simulink model "soc_dvbs2_fpga"  (R2025b)
settings: Solver=FixedStepDiscrete  StartTime=0.0  StopTime=0  RelTol=1e-3
InitFcn:
  | soc_dvbs2_init;
values from neighbouring files (symbols this model uses):
  Rsym = 4e6    (= 4000000)    [soc_dvbs2_init.m]
  soc_dvbs2_txPacketBits = [1 1 0 1 0 1 1 1 0 1 1 1 ... (2972 elements, 2972x1)]    [soc_dvbs2_txPacketBits.mat]
  syncWord = (dec2bin(hex2dec('AC')) - '0').'    [soc_dvbs2_init.m]
  txDataOut = txobj(frameBits(:))    [soc_dvbs2_init.m]
  txFiltCoeff = txobj.pTxFilterCoeff    [soc_dvbs2_init.m]
undefined symbols (not defined in the file or in its folder): Add, coefficientsLog, coefficientsSqrt1, coefficientsSqrt2, dataBits, designMultirateFIR, noisePow, NumBits1, NumBits2, seedsURNG1, seedsURNG2, Shift, Slope1, Slope2, soc_dvbs2_designFIRFilter, txDataOutS1, txDataOutS10, txDataOutS12, txDataOutS13, txDataOutS14, txDataOutS15, txDataOutS16, txDataOutS18, txDataOutS19, txDataOutS2, txDataOutS20, txDataOutS21, txDataOutS22, txDataOutS24, txDataOutS25, txDataOutS26, txDataOutS27, txDataOutS3, txDataOutS4, txDataOutS5, txDataOutS6, txDataOutS7, txDataOutS8, txDataOutS9
libraries: simulink x214, hdlsllib x211, dspsigops x22, dsphdlfiltering2 x8, dsphdlsigops2 x5, commseqgen3 x5, dsphdlmathfun2 x3, hwlogicconnlib x2, whdledac x2, commhdlcrc x2, whdlutilities x1, whdlmod x1
(part 6 of 12)

== system soc_dvbs2_fpga/DVBS2/DVBS2 TxRx/DVB-S2 HDL Receiver/Stream Recovery/BB Decoder/Extract BBHeader/Extract MATYPE1 ==
  bitsIn : Inport
  idx : Inport  Port=2
  validIn : Inport  Port=3
  Bit Concat : hdlsllib/Logic and Bit Operations/Bit Concat  numInputs=2
  Bit Concat1 : hdlsllib/Logic and Bit Operations/Bit Concat  numInputs=2
  Compare To Constant : simulink/Logic and Bit Operations/Compare To Constant  relop===  const=0  OutDataTypeStr=boolean
  Compare To Constant1 : simulink/Logic and Bit Operations/Compare To Constant  relop===  const=1  OutDataTypeStr=boolean
  Compare To Constant2 : simulink/Logic and Bit Operations/Compare To Constant  relop===  const=2  OutDataTypeStr=boolean
  Compare To Constant3 : simulink/Logic and Bit Operations/Compare To Constant  relop===  const=3  OutDataTypeStr=boolean
  Compare To Constant4 : simulink/Logic and Bit Operations/Compare To Constant  relop===  const=4  OutDataTypeStr=boolean
  Compare To Constant5 : simulink/Logic and Bit Operations/Compare To Constant  relop===  const=5  OutDataTypeStr=boolean
  Compare To Constant6 : simulink/Logic and Bit Operations/Compare To Constant  relop===  const=6  OutDataTypeStr=boolean
  Compare To Constant7 : simulink/Logic and Bit Operations/Compare To Constant  relop===  const=7  OutDataTypeStr=boolean
  Delay{,1..6} (7 alike) : Delay  DelayLength=1
  Logical Operator{,1..7} (8 alike) : Logic  AllPortsSameDT=off  OutDataTypeStr=boolean
  Unit Delay Enabled Synchronous{,1..7} (8 alike) : hdlsllib/Discrete/Unit Delay Enabled Synchronous  InitialCondition=0.0  SampleTime=-1
  TSorGS : Outport
  SISorMIS : Outport  Port=2
  CCMorACM : Outport  Port=3
  ISSYI : Outport  Port=4
  NPD : Outport  Port=5
  RO : Outport  Port=6
  wires:
  Delay6/1 -> Unit Delay Enabled Synchronous7/2
  Unit Delay Enabled Synchronous7/1 -> RO/1
  Logical Operator7/1 -> Delay6/1
  Bit Concat1/1 -> Unit Delay Enabled Synchronous7/1
  Unit Delay Enabled Synchronous6/1 -> Bit Concat1/1
  validIn/1 -> Logical Operator/2, Logical Operator3/2, Logical Operator4/2, Logical Operator5/2, Logical Operator6/2, Logical Operator7/2, Logical Operator2/2, Logical Operator1/2
  Compare To Constant7/1 -> Logical Operator7/1
  Compare To Constant6/1 -> Logical Operator6/1
  Logical Operator6/1 -> Unit Delay Enabled Synchronous6/2
  Unit Delay Enabled Synchronous5/1 -> NPD/1
  Delay5/1 -> Unit Delay Enabled Synchronous5/2
  Logical Operator5/1 -> Delay5/1
  Compare To Constant5/1 -> Logical Operator5/1
  Unit Delay Enabled Synchronous1/1 -> TSorGS/1
  Unit Delay Enabled Synchronous4/1 -> ISSYI/1
  Logical Operator/1 -> Unit Delay Enabled Synchronous/2
  Compare To Constant3/1 -> Logical Operator3/1
  Delay/1 -> Unit Delay Enabled Synchronous1/2
  Logical Operator2/1 -> Delay2/1
  Logical Operator3/1 -> Delay3/1
  Compare To Constant/1 -> Logical Operator/1
  Compare To Constant4/1 -> Logical Operator4/1
  Delay2/1 -> Unit Delay Enabled Synchronous2/2
  bitsIn/1 -> Unit Delay Enabled Synchronous/1, Delay1/1, Unit Delay Enabled Synchronous6/1
  Delay4/1 -> Unit Delay Enabled Synchronous4/2
  Delay1/1 -> Bit Concat/2, Unit Delay Enabled Synchronous2/1, Unit Delay Enabled Synchronous3/1, Unit Delay Enabled Synchronous4/1, Unit Delay Enabled Synchronous5/1, Bit Concat1/2
  Bit Concat/1 -> Unit Delay Enabled Synchronous1/1
  Logical Operator4/1 -> Delay4/1
  idx/1 -> Compare To Constant/1, Compare To Constant1/1, Compare To Constant2/1, Compare To Constant3/1, Compare To Constant5/1, Compare To Constant6/1, Compare To Constant7/1, Compare To Constant4/1
  Compare To Constant1/1 -> Logical Operator1/1
  Unit Delay Enabled Synchronous3/1 -> CCMorACM/1
  Logical Operator1/1 -> Delay/1
  Delay3/1 -> Unit Delay Enabled Synchronous3/2
  Unit Delay Enabled Synchronous/1 -> Bit Concat/1
  Unit Delay Enabled Synchronous2/1 -> SISorMIS/1
  Compare To Constant2/1 -> Logical Operator2/1

== system soc_dvbs2_fpga/DVBS2/DVBS2 TxRx/DVB-S2 HDL Receiver/Stream Recovery/BB Decoder/Extract BBHeader/Extract MATYPE2 ==
  bitsIn : Inport
  idx : Inport  Port=2
  validIn : Inport  Port=3
  Add : Sum  Inputs=|++  OutDataTypeStr=Inherit: Same as first input
  Compare To Constant : simulink/Logic and Bit Operations/Compare To Constant  relop=>=  const=8  OutDataTypeStr=boolean
  Compare To Constant1 : simulink/Logic and Bit Operations/Compare To Constant  relop=<=  const=8+7  OutDataTypeStr=boolean
  Compare To Constant2 : simulink/Logic and Bit Operations/Compare To Constant  relop===  const=16  OutDataTypeStr=boolean
  Data Type Conversion : DataTypeConversion  OutDataTypeStr=uint8  SaturateOnIntegerOverflow=off  RndMeth=Floor
  Gain : Gain  Gain=2  ParamDataTypeStr=fixdt(0,2,0)  OutDataTypeStr=Inherit: Same as input
  Logical Operator : Logic  Inputs=3  AllPortsSameDT=off  OutDataTypeStr=boolean
  Logical Operator1 : Logic  AllPortsSameDT=off  OutDataTypeStr=boolean
  Unit Delay Enabled Synchronous : hdlsllib/Discrete/Unit Delay Enabled Synchronous  InitialCondition=0.0  SampleTime=-1
  Unit Delay Enabled Resettable Synchronous : hdlsllib/Discrete/Unit Delay Enabled Resettable Synchronous  InitialCondition=0.0  SampleTime=-1
  MIS_ISI : Outport
  wires:
  bitsIn/1 -> Data Type Conversion/1
  Compare To Constant1/1 -> Logical Operator/2
  Gain/1 -> Add/2
  Unit Delay Enabled Synchronous/1 -> MIS_ISI/1
  Data Type Conversion/1 -> Add/1
  Compare To Constant2/1 -> Logical Operator1/1
  Unit Delay Enabled Resettable Synchronous/1 -> Unit Delay Enabled Synchronous/1, Gain/1
  idx/1 -> Compare To Constant1/1, Compare To Constant2/1, Compare To Constant/1
  Add/1 -> Unit Delay Enabled Resettable Synchronous/1
  Logical Operator/1 -> Unit Delay Enabled Resettable Synchronous/2
  validIn/1 -> Logical Operator1/2, Logical Operator/3
  Logical Operator1/1 -> Unit Delay Enabled Resettable Synchronous/3, Unit Delay Enabled Synchronous/2
  Compare To Constant/1 -> Logical Operator/1

== system soc_dvbs2_fpga/DVBS2/DVBS2 TxRx/DVB-S2 HDL Receiver/Stream Recovery/BB Decoder/Extract BBHeader/Extract SYNC ==
  bitsIn : Inport
  idx : Inport  Port=2
  validIn : Inport  Port=3
  Add : Sum  Inputs=|++  OutDataTypeStr=Inherit: Same as first input
  Compare To Constant : simulink/Logic and Bit Operations/Compare To Constant  relop=>=  const=48  OutDataTypeStr=boolean
  Compare To Constant1 : simulink/Logic and Bit Operations/Compare To Constant  relop=<=  const=48+7  OutDataTypeStr=boolean
  Compare To Constant2 : simulink/Logic and Bit Operations/Compare To Constant  relop===  const=56  OutDataTypeStr=boolean
  Data Type Conversion : DataTypeConversion  OutDataTypeStr=uint8  SaturateOnIntegerOverflow=off  RndMeth=Floor
  Gain : Gain  Gain=2  ParamDataTypeStr=fixdt(0,2,0)  OutDataTypeStr=Inherit: Same as input
  Logical Operator : Logic  Inputs=3  AllPortsSameDT=off  OutDataTypeStr=boolean
  Logical Operator1 : Logic  AllPortsSameDT=off  OutDataTypeStr=boolean
  Unit Delay Enabled Synchronous : hdlsllib/Discrete/Unit Delay Enabled Synchronous  InitialCondition=0.0  SampleTime=-1
  Unit Delay Enabled Resettable Synchronous : hdlsllib/Discrete/Unit Delay Enabled Resettable Synchronous  InitialCondition=0.0  SampleTime=-1
  SYNC : Outport
  wires:
  Compare To Constant/1 -> Logical Operator/1
  Logical Operator1/1 -> Unit Delay Enabled Synchronous/2, Unit Delay Enabled Resettable Synchronous/3
  validIn/1 -> Logical Operator1/2, Logical Operator/3
  Logical Operator/1 -> Unit Delay Enabled Resettable Synchronous/2
  Add/1 -> Unit Delay Enabled Resettable Synchronous/1
  idx/1 -> Compare To Constant2/1, Compare To Constant1/1, Compare To Constant/1
  Unit Delay Enabled Resettable Synchronous/1 -> Gain/1, Unit Delay Enabled Synchronous/1
  Compare To Constant2/1 -> Logical Operator1/1
  Data Type Conversion/1 -> Add/1
  Unit Delay Enabled Synchronous/1 -> SYNC/1
  Gain/1 -> Add/2
  Compare To Constant1/1 -> Logical Operator/2
  bitsIn/1 -> Data Type Conversion/1

== system soc_dvbs2_fpga/DVBS2/DVBS2 TxRx/DVB-S2 HDL Receiver/Stream Recovery/BB Decoder/Extract BBHeader/Extract SYNCD ==
  bitsIn : Inport
  idx : Inport  Port=2
  validIn : Inport  Port=3
  Add : Sum  Inputs=|++  OutDataTypeStr=Inherit: Same as first input
  Compare To Constant : simulink/Logic and Bit Operations/Compare To Constant  relop=>=  const=56  OutDataTypeStr=boolean
  Compare To Constant1 : simulink/Logic and Bit Operations/Compare To Constant  relop=<=  const=56+15  OutDataTypeStr=boolean
  Data Type Conversion : DataTypeConversion  OutDataTypeStr=uint16  SaturateOnIntegerOverflow=off  RndMeth=Floor
  Delay : Delay  DelayLength=1
  Gain : Gain  Gain=2  ParamDataTypeStr=fixdt(0,2,0)  OutDataTypeStr=Inherit: Same as input
  Logical Operator : Logic  Inputs=3  AllPortsSameDT=off  OutDataTypeStr=boolean
  Logical Operator1 : Logic  AllPortsSameDT=off  OutDataTypeStr=boolean
  Unit Delay Enabled Synchronous : hdlsllib/Discrete/Unit Delay Enabled Synchronous  InitialCondition=0.0  SampleTime=-1
  Unit Delay Enabled Resettable Synchronous : hdlsllib/Discrete/Unit Delay Enabled Resettable Synchronous  InitialCondition=0.0  SampleTime=-1
  DFL : Outport
  wires:
  Delay/1 -> Unit Delay Enabled Synchronous/2, Unit Delay Enabled Resettable Synchronous/3
  Compare To Constant/1 -> Logical Operator/1
  Logical Operator1/1 -> Delay/1
  validIn/1 -> Logical Operator1/2, Logical Operator/3
  Logical Operator/1 -> Unit Delay Enabled Resettable Synchronous/2
  Add/1 -> Unit Delay Enabled Resettable Synchronous/1
  idx/1 -> Compare To Constant1/1, Compare To Constant/1
  Unit Delay Enabled Resettable Synchronous/1 -> Gain/1, Unit Delay Enabled Synchronous/1
  Data Type Conversion/1 -> Add/1
  Unit Delay Enabled Synchronous/1 -> DFL/1
  Gain/1 -> Add/2
  Compare To Constant1/1 -> Logical Operator/2, Logical Operator1/1
  bitsIn/1 -> Data Type Conversion/1

== system soc_dvbs2_fpga/DVBS2/DVBS2 TxRx/DVB-S2 HDL Receiver/Stream Recovery/BB Decoder/Extract BBHeader/Extract UPL ==
  bitsIn : Inport
  idx : Inport  Port=2
  validIn : Inport  Port=3
  Add : Sum  Inputs=|++  OutDataTypeStr=Inherit: Same as first input
  Compare To Constant : simulink/Logic and Bit Operations/Compare To Constant  relop=>=  const=16  OutDataTypeStr=boolean
  Compare To Constant1 : simulink/Logic and Bit Operations/Compare To Constant  relop=<=  const=16+15  OutDataTypeStr=boolean
  Compare To Constant2 : simulink/Logic and Bit Operations/Compare To Constant  relop===  const=32  OutDataTypeStr=boolean
  Data Type Conversion : DataTypeConversion  OutDataTypeStr=uint16  SaturateOnIntegerOverflow=off  RndMeth=Floor
  Gain : Gain  Gain=2  ParamDataTypeStr=fixdt(0,2,0)  OutDataTypeStr=Inherit: Same as input
  Logical Operator : Logic  Inputs=3  AllPortsSameDT=off  OutDataTypeStr=boolean
  Logical Operator1 : Logic  AllPortsSameDT=off  OutDataTypeStr=boolean
  Unit Delay Enabled Synchronous : hdlsllib/Discrete/Unit Delay Enabled Synchronous  InitialCondition=0.0  SampleTime=-1
  Unit Delay Enabled Resettable Synchronous : hdlsllib/Discrete/Unit Delay Enabled Resettable Synchronous  InitialCondition=0.0  SampleTime=-1
  UPL : Outport
  wires:
  Compare To Constant/1 -> Logical Operator/1
  Logical Operator1/1 -> Unit Delay Enabled Synchronous/2, Unit Delay Enabled Resettable Synchronous/3
  validIn/1 -> Logical Operator1/2, Logical Operator/3
  Logical Operator/1 -> Unit Delay Enabled Resettable Synchronous/2
  Add/1 -> Unit Delay Enabled Resettable Synchronous/1
  idx/1 -> Compare To Constant2/1, Compare To Constant1/1, Compare To Constant/1
  Unit Delay Enabled Resettable Synchronous/1 -> Gain/1, Unit Delay Enabled Synchronous/1
  Compare To Constant2/1 -> Logical Operator1/1
  Data Type Conversion/1 -> Add/1
  Unit Delay Enabled Synchronous/1 -> UPL/1
  Gain/1 -> Add/2
  Compare To Constant1/1 -> Logical Operator/2
  bitsIn/1 -> Data Type Conversion/1

== system soc_dvbs2_fpga/DVBS2/DVBS2 TxRx/DVB-S2 HDL Receiver/Stream Recovery/BB Decoder/Extract BBHeader/Saturate UPL value ==
  note: if UPL > DFL - 10
      | saturatedUPL = DFL - 10;
      | else
      | saturatedUPL = UPL
      | end
  UPL : Inport
  DFL : Inport  Port=2
  Add : Sum  Inputs=+-  OutDataTypeStr=Inherit: Same as first input
  Constant : Constant  Value=10  OutDataTypeStr=fixdt(0,4,0)  SampleTime=-1
  Relational Operator : RelationalOperator  Operator=>  OutDataTypeStr=boolean  RndMeth=Simplest  InputSameDT=off
  Switch : Switch  Criteria=u2 ~= 0  SaturateOnIntegerOverflow=off  InputSameDT=off
  saturatedUPL : Outport
  wires:
  Constant/1 -> Add/2
  Relational Operator/1 -> Switch/2
  UPL/1 -> Switch/3, Relational Operator/1
  Add/1 -> Relational Operator/2, Switch/1
  DFL/1 -> Add/1
  Switch/1 -> saturatedUPL/1

== system soc_dvbs2_fpga/DVBS2/DVBS2 TxRx/DVB-S2 HDL Receiver/Stream Recovery/BB Decoder/Extract Data Field/Indicate SYNCD bit ==
  rst : Inport
  Distance : Inport  Port=2
  validIn : Inport  Port=3
  Constant1 : Constant  OutDataTypeStr=fixdt(0,1,0)  SampleTime=-1
  Constant2 : Constant  Value=0  OutDataTypeStr=fixdt(0,1,0)  SampleTime=-1
  HDL Counter1 : hdlsllib/Sources/HDL Counter  CountType=Free running  CountInit=0  CountStep=1  CountMax=25  CountFromType=Initial value  CountFrom=0  CountResetPort=on  CountLoadPort=off  CountEnbPort=on  CountDirPort=off  CountHitOutputPort=off  CountDataType=Unsigned  CountWordLen=16  CountFracLen=0  CountSampTime=1
  Logical Operator3 : Logic  AllPortsSameDT=off  OutDataTypeStr=boolean
  Relational Operator1 : RelationalOperator  Operator===  OutDataTypeStr=boolean  RndMeth=Simplest  InputSameDT=off
  Subtract1 : Sum  Inputs=+-  OutDataTypeStr=Inherit: Same as first input
  Switch : Switch  Criteria=u2 ~= 0  SaturateOnIntegerOverflow=off  InputSameDT=off
  trigger : Outport
  wires:
  rst/1 -> HDL Counter1/1
  Logical Operator3/1 -> trigger/1
  Switch/1 -> Subtract1/2
  validIn/1 -> HDL Counter1/2, Logical Operator3/2
  Distance/1 -> Subtract1/1, Switch/2
  Subtract1/1 -> Relational Operator1/1
  Relational Operator1/1 -> Logical Operator3/1
  Constant2/1 -> Switch/3
  Constant1/1 -> Switch/1
  HDL Counter1/1 -> Relational Operator1/2

== system soc_dvbs2_fpga/DVBS2/DVBS2 TxRx/DVB-S2 HDL Receiver/Stream Recovery/BB Decoder/Extract Stream/Extract User Packet  ==
  SYNCD : Inport
  bitsIn : Inport  Port=2
  startIn : Inport  Port=3
  endIn : Inport  Port=4
  validIn : Inport  Port=5
  UPL : Inport  Port=6
  Compare To Constant : simulink/Logic and Bit Operations/Compare To Constant  relop=~=  const=0  OutDataTypeStr=boolean
  Delay{1..2,4..7,9..10,12,19,21} (11 alike) : Delay  DelayLength=1
  Demux : Demux  Outputs=2
  Indicate SYNCD bit : Subsystem
  Logical Operator : Logic  AllPortsSameDT=off  OutDataTypeStr=boolean
  Logical Operator1 : Logic  AllPortsSameDT=off  OutDataTypeStr=boolean
  Logical Operator2 : Logic  Operator=NOT  AllPortsSameDT=off  OutDataTypeStr=boolean
  Logical Operator3 : Logic  Operator=OR  AllPortsSameDT=off  OutDataTypeStr=boolean
  Sample Discard Control : MATLAB Function  TreatAsAtomicUnit=on
  Terminator1 : Terminator
  Variable Count Limited HDL Counter : MATLAB Function  TreatAsAtomicUnit=on
  dataOut : Outport
  startOut : Outport  Port=2
  endOut : Outport  Port=3
  validOut : Outport  Port=4
  invalidPkt : Outport  Port=5
  wires:
  validIn/1 -> Logical Operator/2
  Compare To Constant/1 -> Logical Operator/1
  Demux/2 -> Logical Operator2/1, Logical Operator3/1
  Demux/1 -> startOut/1
  Delay12/1 -> Sample Discard Control/2(startIn)
  Delay10/1 -> dataOut/1
  Delay9/1 -> Sample Discard Control/3(endIn)
  Variable Count Limited HDL Counter/1(Hit) -> Sample Discard Control/1(dataIn)
  Delay21/1 -> Delay6/1
  Logical Operator/1 -> Delay2/1
  UPL/1 -> Delay21/1, Compare To Constant/1
  Delay5/1 -> Sample Discard Control/4(validIn), Variable Count Limited HDL Counter/3(enb)
  Delay6/1 -> Variable Count Limited HDL Counter/2(countToValue)
  Delay7/1 -> Delay9/1
  endIn/1 -> Delay7/1
  Indicate SYNCD bit/1(trigger) -> Delay12/1, Variable Count Limited HDL Counter/1(rst)
  startIn/1 -> Indicate SYNCD bit/1(rst)
  Delay1/1 -> Indicate SYNCD bit/2(Distance)
  Delay4/1 -> Delay10/1
  SYNCD/1 -> Delay1/1
  Delay2/1 -> Delay5/1, Indicate SYNCD bit/3(validIn)
  bitsIn/1 -> Delay19/1
  Delay19/1 -> Delay4/1
  Sample Discard Control/1(dataOut) -> Demux/1
  Sample Discard Control/2(startOut) -> Terminator1/1
  Sample Discard Control/3(endOut) -> Logical Operator3/2, Logical Operator1/2
  Sample Discard Control/4(validOut) -> validOut/1
  Logical Operator1/1 -> invalidPkt/1
  Logical Operator2/1 -> Logical Operator1/1
  Logical Operator3/1 -> endOut/1

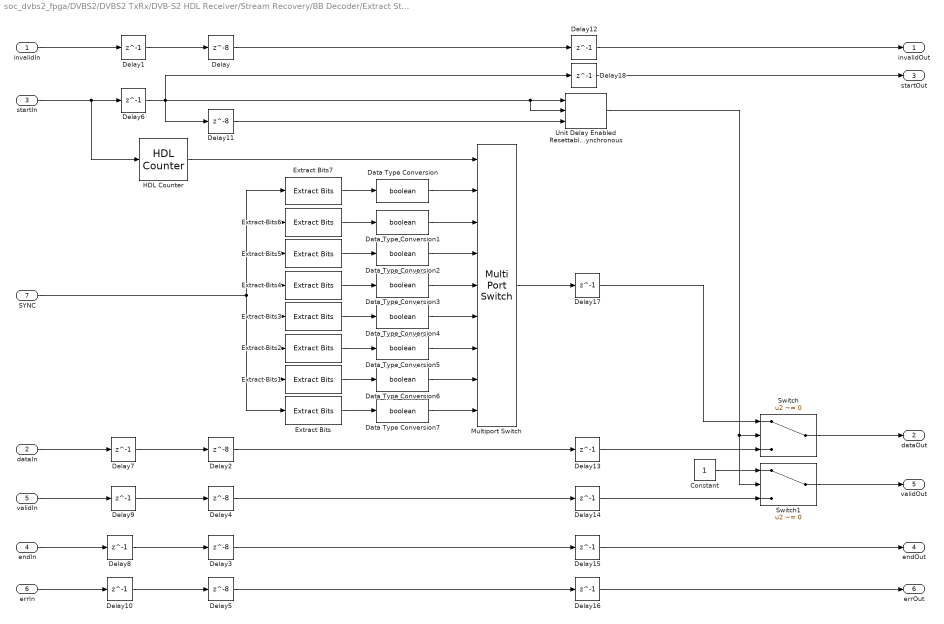
== system soc_dvbs2_fpga/DVBS2/DVBS2 TxRx/DVB-S2 HDL Receiver/Stream Recovery/BB Decoder/Extract Stream/Insert SYNC ==
  invalidIn : Inport
  dataIn : Inport  Port=2
  startIn : Inport  Port=3
  endIn : Inport  Port=4
  validIn : Inport  Port=5
  errIn : Inport  Port=6
  SYNC : Inport  Port=7
  Constant : Constant  OutDataTypeStr=boolean  SampleTime=-1
  Data Type Conversion{,1..7} (8 alike) : DataTypeConversion  OutDataTypeStr=boolean  SaturateOnIntegerOverflow=off  RndMeth=Floor
  Delay{,2..5,11} (6 alike) : Delay  DelayLength=8
  Delay{1,6..10,12..18} (13 alike) : Delay  DelayLength=1
  Extract Bits : simulink/Logic and Bit Operations/Extract Bits  bitsToExtract=Range of bits  numBits=8  bitIdxRange=0  outScalingMode=Treat bit field as an integer
  Extract Bits1 : simulink/Logic and Bit Operations/Extract Bits  bitsToExtract=Range of bits  numBits=8  bitIdxRange=1  outScalingMode=Treat bit field as an integer
  Extract Bits2 : simulink/Logic and Bit Operations/Extract Bits  bitsToExtract=Range of bits  numBits=8  bitIdxRange=2  outScalingMode=Treat bit field as an integer
  Extract Bits3 : simulink/Logic and Bit Operations/Extract Bits  bitsToExtract=Range of bits  numBits=8  bitIdxRange=3  outScalingMode=Treat bit field as an integer
  Extract Bits4 : simulink/Logic and Bit Operations/Extract Bits  bitsToExtract=Range of bits  numBits=8  bitIdxRange=4  outScalingMode=Treat bit field as an integer
  Extract Bits5 : simulink/Logic and Bit Operations/Extract Bits  bitsToExtract=Range of bits  numBits=8  bitIdxRange=5  outScalingMode=Treat bit field as an integer
  Extract Bits6 : simulink/Logic and Bit Operations/Extract Bits  bitsToExtract=Range of bits  numBits=8  bitIdxRange=6  outScalingMode=Treat bit field as an integer
  Extract Bits7 : simulink/Logic and Bit Operations/Extract Bits  bitsToExtract=Range of bits  numBits=8  bitIdxRange=7  outScalingMode=Treat bit field as an integer
  HDL Counter : hdlsllib/Sources/HDL Counter  CountType=Count limited  CountInit=0  CountStep=1  CountMax=7  CountFromType=Initial value  CountFrom=0  CountResetPort=on  CountLoadPort=off  CountEnbPort=off  CountDirPort=off  CountHitOutputPort=off  CountDataType=Unsigned  CountWordLen=3  CountFracLen=0  CountSampTime=1
  Multiport Switch : MultiPortSwitch  DataPortOrder=Zero-based contiguous  Inputs=8  zeroidx=on  SaturateOnIntegerOverflow=off  InputSameDT=off
  Switch : Switch  Criteria=u2 ~= 0  SaturateOnIntegerOverflow=off  InputSameDT=off
  Switch1 : Switch  Criteria=u2 ~= 0  SaturateOnIntegerOverflow=off  InputSameDT=off
  Unit Delay Enabled Resettable Synchronous : hdlsllib/Discrete/Unit Delay Enabled Resettable Synchronous  InitialCondition=0.0  SampleTime=-1
  invalidOut : Outport
  dataOut : Outport  Port=2
  startOut : Outport  Port=3
  endOut : Outport  Port=4
  validOut : Outport  Port=5
  errOut : Outport  Port=6
  wires:
  Switch/1 -> dataOut/1
  Switch1/1 -> validOut/1
  Delay18/1 -> startOut/1
  Delay10/1 -> Delay5/1
  errIn/1 -> Delay10/1
  endIn/1 -> Delay8/1
  Delay14/1 -> Switch1/3
  Data Type Conversion7/1 -> Multiport Switch/9
  Multiport Switch/1 -> Delay17/1
  startIn/1 -> HDL Counter/1, Delay6/1
  Delay2/1 -> Delay13/1
  Delay12/1 -> invalidOut/1
  Data Type Conversion1/1 -> Multiport Switch/3
  Extract Bits4/1 -> Data Type Conversion3/1
  Unit Delay Enabled Resettable Synchronous/1 -> Switch1/2, Switch/2
  Delay6/1 -> Delay18/1, Delay11/1, Unit Delay Enabled Resettable Synchronous/2, Unit Delay Enabled Resettable Synchronous/1
  Data Type Conversion5/1 -> Multiport Switch/7
  Delay1/1 -> Delay/1
  Extract Bits/1 -> Data Type Conversion7/1
  dataIn/1 -> Delay7/1
  Delay7/1 -> Delay2/1
  Delay11/1 -> Unit Delay Enabled Resettable Synchronous/3
  Extract Bits1/1 -> Data Type Conversion6/1
  invalidIn/1 -> Delay1/1
  Delay9/1 -> Delay4/1
  Extract Bits6/1 -> Data Type Conversion1/1
  Data Type Conversion4/1 -> Multiport Switch/6
  Data Type Conversion2/1 -> Multiport Switch/4
  Data Type Conversion3/1 -> Multiport Switch/5
  Extract Bits5/1 -> Data Type Conversion2/1
  Extract Bits7/1 -> Data Type Conversion/1
  Delay5/1 -> Delay16/1
  Data Type Conversion6/1 -> Multiport Switch/8
  Delay16/1 -> errOut/1
  Delay17/1 -> Switch/1
  validIn/1 -> Delay9/1
  HDL Counter/1 -> Multiport Switch/1
  Constant/1 -> Switch1/1
  Delay3/1 -> Delay15/1
  Delay8/1 -> Delay3/1
  Delay/1 -> Delay12/1
  Extract Bits2/1 -> Data Type Conversion5/1
  Delay13/1 -> Switch/3
  Delay15/1 -> endOut/1
  Data Type Conversion/1 -> Multiport Switch/2
  Extract Bits3/1 -> Data Type Conversion4/1
  SYNC/1 -> Extract Bits7/1, Extract Bits6/1, Extract Bits5/1, Extract Bits4/1, Extract Bits/1, Extract Bits1/1, Extract Bits2/1, Extract Bits3/1
  Delay4/1 -> Delay14/1

== system soc_dvbs2_fpga/DVBS2/DVBS2 TxRx/DVB-S2 HDL Receiver/Synchronizer and PL Header Decoder/Fine Phase Synchronizer/Power Q and Beta Offset Rotation/Complex Multiplier ==
  In1 : Inport
  In2 : Inport  Port=2
  AddADn : Sum  Inputs=++|  OutDataTypeStr=Inherit: Inherit via back propagation
  AddAUp : Sum  Inputs=|+-  OutDataTypeStr=Inherit: Inherit via back propagation
  AddBCtr : Sum  Inputs=+|+
  AddBDn : Sum  Inputs=|+-
  AddBUp : Sum  Inputs=++|
  Complex to Real-Imag : ComplexToRealImag
  Complex to Real-Imag1 : ComplexToRealImag
  Data Type Duplicate : DataTypeDuplicate
  Delay{1..8,21} (9 alike) : Delay
  Delay{9..20} (12 alike) : Delay  DelayLength=1
  ProductCtr : Product
  ProductDn : Product
  ProductUp : Product
  Real-Imag to Complex : RealImagToComplex
  Out1 : Outport  VectorParamsAs1DForOutWhenUnconnected=off
  wires:
  In1/1 -> Complex to Real-Imag/1, Data Type Duplicate/1
  In2/1 -> Complex to Real-Imag1/1
  Complex to Real-Imag1/1 -> [RE2]
  Complex to Real-Imag1/2 -> [IM2]
  [IM2] -> Delay10/1
  [RE2] -> Delay9/1
  Complex to Real-Imag/1 -> Delay11/1
  AddBUp/1 -> Delay8/1
  [RE2] -> Delay14/1
  [IM2] -> Delay15/1
  AddBDn/1 -> Delay5/1
  Complex to Real-Imag/2 -> Delay13/1
  AddBCtr/1 -> Delay2/1
  [IM2] -> Delay12/1
  ProductUp/1 -> Delay21/1
  ProductCtr/1 -> Delay7/1
  ProductDn/1 -> Delay6/1
  AddADn/1 -> Delay20/1
  AddAUp/1 -> Delay19/1
  Real-Imag to Complex/1 -> Out1/1, Data Type Duplicate/2
  Delay21/1 -> Delay16/1
  Delay7/1 -> Delay17/1
  Delay6/1 -> Delay18/1
  Delay5/1 -> ProductDn/2
  Delay4/1 -> ProductDn/1
  Delay3/1 -> ProductCtr/2
  Delay2/1 -> ProductCtr/1
  Delay1/1 -> ProductUp/2
  Delay8/1 -> ProductUp/1
  Delay9/1 -> AddBUp/1
  Delay10/1 -> AddBUp/2
  Delay11/1 -> Delay1/1, AddBCtr/1
  Delay12/1 -> Delay3/1
  Delay13/1 -> Delay4/1, AddBCtr/2
  Delay14/1 -> AddBDn/1
  Delay15/1 -> AddBDn/2
  Delay16/1 -> AddAUp/1
  Delay17/1 -> AddADn/1, AddAUp/2
  Delay18/1 -> AddADn/2
  Delay19/1 -> Real-Imag to Complex/1
  Delay20/1 -> Real-Imag to Complex/2

== system soc_dvbs2_fpga/DVBS2/DVBS2 TxRx/DVB-S2 HDL Receiver/Synchronizer and PL Header Decoder/Fine Phase Synchronizer/Power Q and Beta Offset Rotation/Complex Multiplier1 ==
  In1 : Inport
  In2 : Inport  Port=2
  AddADn : Sum  Inputs=++|  OutDataTypeStr=Inherit: Inherit via back propagation
  AddAUp : Sum  Inputs=|+-  OutDataTypeStr=Inherit: Inherit via back propagation
  AddBCtr : Sum  Inputs=+|+
  AddBDn : Sum  Inputs=|+-
  AddBUp : Sum  Inputs=++|
  Complex to Real-Imag : ComplexToRealImag
  Complex to Real-Imag1 : ComplexToRealImag
  Data Type Duplicate : DataTypeDuplicate
  Delay{1..8,21} (9 alike) : Delay
  Delay{9..20} (12 alike) : Delay  DelayLength=1
  ProductCtr : Product
  ProductDn : Product
  ProductUp : Product
  Real-Imag to Complex : RealImagToComplex
  Out1 : Outport  VectorParamsAs1DForOutWhenUnconnected=off
  wires:
  Delay20/1 -> Real-Imag to Complex/2
  Delay19/1 -> Real-Imag to Complex/1
  Delay18/1 -> AddADn/2
  Delay17/1 -> AddAUp/2, AddADn/1
  Delay16/1 -> AddAUp/1
  Delay15/1 -> AddBDn/2
  Delay14/1 -> AddBDn/1
  Delay13/1 -> AddBCtr/2, Delay4/1
  Delay12/1 -> Delay3/1
  Delay11/1 -> AddBCtr/1, Delay1/1
  Delay10/1 -> AddBUp/2
  Delay9/1 -> AddBUp/1
  Delay8/1 -> ProductUp/1
  Delay1/1 -> ProductUp/2
  Delay2/1 -> ProductCtr/1
  Delay3/1 -> ProductCtr/2
  Delay4/1 -> ProductDn/1
  Delay5/1 -> ProductDn/2
  Delay6/1 -> Delay18/1
  Delay7/1 -> Delay17/1
  Delay21/1 -> Delay16/1
  Real-Imag to Complex/1 -> Data Type Duplicate/2, Out1/1
  AddAUp/1 -> Delay19/1
  AddADn/1 -> Delay20/1
  ProductDn/1 -> Delay6/1
  ProductCtr/1 -> Delay7/1
  ProductUp/1 -> Delay21/1
  [IM2] -> Delay12/1
  AddBCtr/1 -> Delay2/1
  Complex to Real-Imag/2 -> Delay13/1
  AddBDn/1 -> Delay5/1
  [IM2] -> Delay15/1
  [RE2] -> Delay14/1
  AddBUp/1 -> Delay8/1
  Complex to Real-Imag/1 -> Delay11/1
  [RE2] -> Delay9/1
  [IM2] -> Delay10/1
  Complex to Real-Imag1/2 -> [IM2]
  Complex to Real-Imag1/1 -> [RE2]
  In2/1 -> Complex to Real-Imag1/1
  In1/1 -> Data Type Duplicate/1, Complex to Real-Imag/1

== system soc_dvbs2_fpga/DVBS2/DVBS2 TxRx/DVB-S2 HDL Receiver/Synchronizer and PL Header Decoder/Fine Phase Synchronizer/Power Q and Beta Offset Rotation/Complex Multiplier2 ==
  In1 : Inport
  In2 : Inport  Port=2
  AddADn : Sum  Inputs=++|  OutDataTypeStr=Inherit: Inherit via back propagation
  AddAUp : Sum  Inputs=|+-  OutDataTypeStr=Inherit: Inherit via back propagation
  AddBCtr : Sum  Inputs=+|+
  AddBDn : Sum  Inputs=|+-
  AddBUp : Sum  Inputs=++|
  Complex to Real-Imag : ComplexToRealImag
  Complex to Real-Imag1 : ComplexToRealImag
  Data Type Duplicate : DataTypeDuplicate
  Delay{1..8,21} (9 alike) : Delay
  Delay{9..20} (12 alike) : Delay  DelayLength=1
  ProductCtr : Product
  ProductDn : Product
  ProductUp : Product
  Real-Imag to Complex : RealImagToComplex
  Out1 : Outport  VectorParamsAs1DForOutWhenUnconnected=off
  wires:
  In1/1 -> Complex to Real-Imag/1, Data Type Duplicate/1
  In2/1 -> Complex to Real-Imag1/1
  Complex to Real-Imag1/1 -> [RE2]
  Complex to Real-Imag1/2 -> [IM2]
  [IM2] -> Delay10/1
  [RE2] -> Delay9/1
  Complex to Real-Imag/1 -> Delay11/1
  AddBUp/1 -> Delay8/1
  [RE2] -> Delay14/1
  [IM2] -> Delay15/1
  AddBDn/1 -> Delay5/1
  Complex to Real-Imag/2 -> Delay13/1
  AddBCtr/1 -> Delay2/1
  [IM2] -> Delay12/1
  ProductUp/1 -> Delay21/1
  ProductCtr/1 -> Delay7/1
  ProductDn/1 -> Delay6/1
  AddADn/1 -> Delay20/1
  AddAUp/1 -> Delay19/1
  Real-Imag to Complex/1 -> Out1/1, Data Type Duplicate/2
  Delay21/1 -> Delay16/1
  Delay7/1 -> Delay17/1
  Delay6/1 -> Delay18/1
  Delay5/1 -> ProductDn/2
  Delay4/1 -> ProductDn/1
  Delay3/1 -> ProductCtr/2
  Delay2/1 -> ProductCtr/1
  Delay1/1 -> ProductUp/2
  Delay8/1 -> ProductUp/1
  Delay9/1 -> AddBUp/1
  Delay10/1 -> AddBUp/2
  Delay11/1 -> Delay1/1, AddBCtr/1
  Delay12/1 -> Delay3/1
  Delay13/1 -> Delay4/1, AddBCtr/2
  Delay14/1 -> AddBDn/1
  Delay15/1 -> AddBDn/2
  Delay16/1 -> AddAUp/1
  Delay17/1 -> AddADn/1, AddAUp/2
  Delay18/1 -> AddADn/2
  Delay19/1 -> Real-Imag to Complex/1
  Delay20/1 -> Real-Imag to Complex/2

== system soc_dvbs2_fpga/DVBS2/DVBS2 TxRx/DVB-S2 HDL Receiver/Synchronizer and PL Header Decoder/Fine Phase Synchronizer/Power Q and Beta Offset Rotation/Gain ==
  In1 : Inport
  AddADn : Sum  Inputs=++|  OutDataTypeStr=Inherit: Inherit via back propagation
  AddAUp : Sum  Inputs=|+-  OutDataTypeStr=Inherit: Inherit via back propagation
  AddBCtr : Sum  Inputs=+|+
  AddBDn : Sum  Inputs=|+-
  AddBUp : Sum  Inputs=++|
  Complex to Real-Imag : ComplexToRealImag
  Complex to Real-Imag1 : ComplexToRealImag
  Constant : Constant  Value=fi(exp(1i*pi/4),1,16)  SampleTime=-1
  Data Type Duplicate : DataTypeDuplicate
  Delay{1..8,21} (9 alike) : Delay
  Delay{9..20} (12 alike) : Delay  DelayLength=1
  ProductCtr : Product
  ProductDn : Product
  ProductUp : Product
  Real-Imag to Complex : RealImagToComplex
  Out1 : Outport  VectorParamsAs1DForOutWhenUnconnected=off
  wires:
  Delay20/1 -> Real-Imag to Complex/2
  Delay19/1 -> Real-Imag to Complex/1
  Delay18/1 -> AddADn/2
  Delay17/1 -> AddAUp/2, AddADn/1
  Delay16/1 -> AddAUp/1
  Delay15/1 -> AddBDn/2
  Delay14/1 -> AddBDn/1
  Delay13/1 -> AddBCtr/2, Delay4/1
  Delay12/1 -> Delay3/1
  Delay11/1 -> AddBCtr/1, Delay1/1
  Delay10/1 -> AddBUp/2
  Delay9/1 -> AddBUp/1
  Delay8/1 -> ProductUp/1
  Delay1/1 -> ProductUp/2
  Delay2/1 -> ProductCtr/1
  Delay3/1 -> ProductCtr/2
  Delay4/1 -> ProductDn/1
  Delay5/1 -> ProductDn/2
  Delay6/1 -> Delay18/1
  Delay7/1 -> Delay17/1
  Delay21/1 -> Delay16/1
  Real-Imag to Complex/1 -> Data Type Duplicate/2, Out1/1
  AddAUp/1 -> Delay19/1
  AddADn/1 -> Delay20/1
  ProductDn/1 -> Delay6/1
  ProductCtr/1 -> Delay7/1
  ProductUp/1 -> Delay21/1
  [IM2] -> Delay12/1
  AddBCtr/1 -> Delay2/1
  Complex to Real-Imag/2 -> Delay13/1
  AddBDn/1 -> Delay5/1
  [IM2] -> Delay15/1
  [RE2] -> Delay14/1
  AddBUp/1 -> Delay8/1
  Complex to Real-Imag/1 -> Delay11/1
  [RE2] -> Delay9/1
  [IM2] -> Delay10/1
  Complex to Real-Imag1/2 -> [IM2]
  Complex to Real-Imag1/1 -> [RE2]
  Constant/1 -> Complex to Real-Imag1/1
  In1/1 -> Data Type Duplicate/1, Complex to Real-Imag/1

== system soc_dvbs2_fpga/DVBS2/DVBS2 TxRx/DVB-S2 HDL Receiver/Synchronizer and PL Header Decoder/Fine Phase Synchronizer/Power Q and Beta Offset Rotation/Gain1 ==
  In1 : Inport
  AddADn : Sum  Inputs=++|  OutDataTypeStr=Inherit: Inherit via back propagation
  AddAUp : Sum  Inputs=|+-  OutDataTypeStr=Inherit: Inherit via back propagation
  AddBCtr : Sum  Inputs=+|+
  AddBDn : Sum  Inputs=|+-
  AddBUp : Sum  Inputs=++|
  Complex to Real-Imag : ComplexToRealImag
  Complex to Real-Imag1 : ComplexToRealImag
  Constant : Constant  Value=fi(exp(1i*pi/4),1,16)  SampleTime=-1
  Data Type Duplicate : DataTypeDuplicate
  Delay{1..8,21} (9 alike) : Delay
  Delay{9..20} (12 alike) : Delay  DelayLength=1
  ProductCtr : Product
  ProductDn : Product
  ProductUp : Product
  Real-Imag to Complex : RealImagToComplex
  Out1 : Outport  VectorParamsAs1DForOutWhenUnconnected=off
  wires:
  In1/1 -> Complex to Real-Imag/1, Data Type Duplicate/1
  Constant/1 -> Complex to Real-Imag1/1
  Complex to Real-Imag1/1 -> [RE2]
  Complex to Real-Imag1/2 -> [IM2]
  [IM2] -> Delay10/1
  [RE2] -> Delay9/1
  Complex to Real-Imag/1 -> Delay11/1
  AddBUp/1 -> Delay8/1
  [RE2] -> Delay14/1
  [IM2] -> Delay15/1
  AddBDn/1 -> Delay5/1
  Complex to Real-Imag/2 -> Delay13/1
  AddBCtr/1 -> Delay2/1
  [IM2] -> Delay12/1
  ProductUp/1 -> Delay21/1
  ProductCtr/1 -> Delay7/1
  ProductDn/1 -> Delay6/1
  AddADn/1 -> Delay20/1
  AddAUp/1 -> Delay19/1
  Real-Imag to Complex/1 -> Out1/1, Data Type Duplicate/2
  Delay21/1 -> Delay16/1
  Delay7/1 -> Delay17/1
  Delay6/1 -> Delay18/1
  Delay5/1 -> ProductDn/2
  Delay4/1 -> ProductDn/1
  Delay3/1 -> ProductCtr/2
  Delay2/1 -> ProductCtr/1
  Delay1/1 -> ProductUp/2
  Delay8/1 -> ProductUp/1
  Delay9/1 -> AddBUp/1
  Delay10/1 -> AddBUp/2
  Delay11/1 -> Delay1/1, AddBCtr/1
  Delay12/1 -> Delay3/1
  Delay13/1 -> Delay4/1, AddBCtr/2
  Delay14/1 -> AddBDn/1
  Delay15/1 -> AddBDn/2
  Delay16/1 -> AddAUp/1
  Delay17/1 -> AddADn/1, AddAUp/2
  Delay18/1 -> AddADn/2
  Delay19/1 -> Real-Imag to Complex/1
  Delay20/1 -> Real-Imag to Complex/2

== system soc_dvbs2_fpga/DVBS2/DVBS2 TxRx/DVB-S2 HDL Receiver/Synchronizer and PL Header Decoder/PL Header Recovery/No HDL1/Subsystem ==
  In1 : Inport
  Enable : EnablePort
  To Workspace5 : ToWorkspace  VariableName=simXFecSampleCount  SaveFormat=Timeseries  SampleTime=-1
      settings: Save2DSignal=2-D array (concatenate along first dimension)
  wires:
  In1/1 -> To Workspace5/1

== system soc_dvbs2_fpga/DVBS2/DVBS2 TxRx/DVB-S2 HDL Receiver/Synchronizer and PL Header Decoder/PL Header Recovery/PL Header Decoder/Bit Flipping and Averaging ==
  dataIn : Inport
  indexIndicater : Inport  Port=2
  validIn : Inport  Port=3
  resetIn : Inport  Port=4
  hasPilots : Inport  Port=5
  Add : Sum  OutDataTypeStr=Inherit: Same as first input
  Delay{1..14} (14 alike) : Delay
  Delay{15..23} (9 alike) : Delay  DelayLength=1
  Gain : Gain  Gain=1/2  ParamDataTypeStr=fixdt(0,1,1)  OutDataTypeStr=Inherit: Same as input
  Gain1 : Gain  Gain=-1  ParamDataTypeStr=fixdt(1,2,0)  OutDataTypeStr=Inherit: Same as input
  Logical Operator : Logic  AllPortsSameDT=off  OutDataTypeStr=boolean
  Logical Operator1 : Logic  AllPortsSameDT=off  OutDataTypeStr=boolean
  Logical Operator2 : Logic  Operator=NOT  AllPortsSameDT=off  OutDataTypeStr=boolean
  Switch1 : Switch  Criteria=u2 ~= 0  SaturateOnIntegerOverflow=off  InputSameDT=off
  Switch2 : Switch  Criteria=u2 ~= 0  SaturateOnIntegerOverflow=off  InputSameDT=off
  Unit Delay Enabled Synchronous : hdlsllib/Discrete/Unit Delay Enabled Synchronous  InitialCondition=0.0  SampleTime=-1
  dataOut : Outport
  validOut : Outport  Port=2
  resetOut : Outport  Port=3
  wires:
  Delay21/1 -> dataOut/1
  Delay23/1 -> resetOut/1
  Delay22/1 -> validOut/1
  Delay20/1 -> Delay23/1
  Delay19/1 -> Logical Operator/2, Logical Operator1/2
  Delay18/1 -> Logical Operator/1, Logical Operator2/1
  Delay17/1 -> Switch2/3
  Delay16/1 -> Switch2/2
  Delay15/1 -> Switch2/1
  Delay14/1 -> Delay20/1
  Delay13/1 -> Delay19/1
  Delay12/1 -> Delay18/1
  Delay11/1 -> Delay14/1
  Delay10/1 -> Delay13/1
  Delay9/1 -> Delay12/1
  Delay8/1 -> Delay16/1
  Delay7/1 -> Delay8/1
  Delay6/1 -> Delay5/1
  Delay5/1 -> Switch1/2
  Delay4/1 -> Delay2/1
  Delay2/1 -> Switch1/3, Delay17/1
  Delay1/1 -> Switch1/1
  Delay3/1 -> Gain1/1
  resetIn/1 -> Delay11/1
  Switch2/1 -> Gain/1
  Add/1 -> Delay21/1
  Logical Operator/1 -> Delay22/1
  Unit Delay Enabled Synchronous/1 -> Add/2
  Gain/1 -> Unit Delay Enabled Synchronous/1, Add/1
  Logical Operator1/1 -> Unit Delay Enabled Synchronous/2
  Logical Operator2/1 -> Logical Operator1/1
  validIn/1 -> Delay10/1
  indexIndicater/1 -> Delay6/1, Delay9/1
  Switch1/1 -> Delay15/1
  hasPilots/1 -> Delay7/1
  dataIn/1 -> Delay4/1, Delay3/1
  Gain1/1 -> Delay1/1

== system soc_dvbs2_fpga/DVBS2/DVBS2 TxRx/DVB-S2 HDL Receiver/Synchronizer and PL Header Decoder/PL Header Recovery/PL Header Decoder/ML Decoder ==
  dataIn : Inport
  PLSCValid32 : Inport  Port=2
  reset : Inport  Port=3
  Code Word LUT 1 to 32 : LookupNDDirect  NumberOfTableDimensions=1  Table=config.intColAllCodeWords1to32
  Code Word LUT 33 to 64 : LookupNDDirect  NumberOfTableDimensions=1  Table=config.intColAllCodeWords33to64
  Compute Euclidean Distance : Subsystem
  Data Type Conversion1 : DataTypeConversion  OutDataTypeStr=fixdt(1,25,15)  SaturateOnIntegerOverflow=off  RndMeth=Floor
  Delay{,15..19} (6 alike) : Delay  DelayLength=1
  Delay{1..2,8..14} (9 alike) : Delay
  Euclidean Distance Sum Up : Subsystem  TreatAsAtomicUnit=on
  Get Min Index : Subsystem
  HDL Counter : hdlsllib/Sources/HDL Counter  CountType=Count limited  CountInit=0  CountStep=1  CountMax=length(config.intColAllCodeWords1to32)-1  CountFromType=Initial value  CountFrom=0  CountResetPort=on  CountLoadPort=off  CountEnbPort=on  CountDirPort=off  CountHitOutputPort=off  CountDataType=Unsigned  CountWordLen=nextpow2(length(config.intColAllCodeWords1to32)-1)  CountFracLen=0  CountSampTime=1
  Integer to Bit Convertor : Subsystem
  Terminator : Terminator
  bits6Out : Outport
  wires:
  Data Type Conversion1/1 -> Delay19/1
  dataIn/1 -> Compute Euclidean Distance/1(softBit)
  Delay2/1 -> Integer to Bit Convertor/2(LS)
  Delay1/1 -> Code Word LUT 33 to 64/1
  Code Word LUT 33 to 64/1 -> Delay2/1
  Compute Euclidean Distance/2(forBit1) -> Delay18/1
  Compute Euclidean Distance/1(forBit0) -> Data Type Conversion1/1
  Delay19/1 -> Euclidean Distance Sum Up/1(Ed0)
  Delay18/1 -> Euclidean Distance Sum Up/2(Ed1)
  Delay17/1 -> Euclidean Distance Sum Up/3(reset)
  Delay16/1 -> Euclidean Distance Sum Up/4(CWswitch)
  Delay15/1 -> Delay8/1, Euclidean Distance Sum Up/5(validIn)
  Delay14/1 -> Delay15/1
  Delay13/1 -> Delay14/1
  Delay12/1 -> Delay17/1
  Delay11/1 -> Delay12/1
  Delay10/1 -> Integer to Bit Convertor/1(MS)
  Delay9/1 -> Code Word LUT 1 to 32/1
  Delay8/1 -> Delay/1
  Get Min Index/2(validOut) -> Terminator/1
  Get Min Index/1(out) -> bits6Out/1
  Euclidean Distance Sum Up/1(CwEdMetric) -> Get Min Index/1(dataIn)
  Delay/1 -> Get Min Index/2(validIn)
  Integer to Bit Convertor/1(Out1) -> Delay16/1
  Code Word LUT 1 to 32/1 -> Delay10/1
  HDL Counter/1 -> Delay1/1, Delay9/1
  reset/1 -> HDL Counter/1, Delay11/1
  PLSCValid32/1 -> HDL Counter/2, Delay13/1

== system soc_dvbs2_fpga/DVBS2/DVBS2 TxRx/DVB-S2 HDL Receiver/Synchronizer and PL Header Decoder/PL Header Recovery/PL Header Decoder/PLSC Descrambler ==
  dataIn : Inport
  resetIn : Inport  Port=2
  validIn : Inport  Port=3
  1-D Lookup Table : Lookup_n-D  NumberOfTableDimensions=1  LookupTableObject=''  BreakpointsSpecification=Even spacing  BreakpointsForDimension1=[-5:5]  BreakpointsForDimension1FirstPoint=0  BreakpointsForDimension2FirstPoint=10  BreakpointsForDimension2Spacing=12  IndexSearchMethod=Evenly spaced points  Table=config.PLSCDescramLUT  TableDataTypeStr=Inherit: Inherit from 'Table data'  InterpMethod=Flat  DiagnosticForOutOfRangeInput=Error  InternalRulePriority=Speed  OutDataTypeStr=Inherit: Inherit from 'Table data'  RndMeth=Simplest
  Data Type Conversion : DataTypeConversion  OutDataTypeStr=boolean  SaturateOnIntegerOverflow=off  RndMeth=Floor
  Delay{1..8} (8 alike) : Delay  DelayLength=1
  Delay{9..27} (19 alike) : Delay
  Extract Bits : simulink/Logic and Bit Operations/Extract Bits  bitsToExtract=Range of bits  numBits=8  bitIdxRange=0  outScalingMode=Preserve fixed-point scaling
  Math Function : Math  Operator=conj
  PLSC Valid Counter : hdlsllib/Sources/HDL Counter  CountType=Count limited  CountInit=0  CountStep=1  CountMax=length(config.PLSCDescramLUT)-1  CountFromType=Initial value  CountFrom=0  CountResetPort=on  CountLoadPort=off  CountEnbPort=on  CountDirPort=off  CountHitOutputPort=off  CountDataType=Unsigned  CountWordLen=nextpow2(length(config.PLSCDescramLUT)-1)  CountFracLen=0  CountSampTime=1
  Product : Product  OutDataTypeStr=Inherit: Same as first input
  dataOut : Outport
  indexIndicator : Outport  Port=2
  validOut : Outport  Port=3
  resetOut : Outport  Port=4
  wires:
  Delay27/1 -> resetOut/1
  Delay26/1 -> validOut/1
  Delay25/1 -> indexIndicator/1
  Delay24/1 -> Delay27/1
  Delay23/1 -> Delay26/1
  Delay22/1 -> Data Type Conversion/1
  Delay21/1 -> dataOut/1
  Delay20/1 -> Product/1
  Delay19/1 -> Product/2
  Delay18/1 -> Delay24/1
  Delay17/1 -> Delay23/1
  Delay16/1 -> Delay22/1
  Delay15/1 -> Delay20/1
  Delay14/1 -> Delay18/1
  Delay13/1 -> Delay17/1
  Delay12/1 -> Extract Bits/1
  Delay11/1 -> Delay15/1
  Delay10/1 -> Math Function/1
  Delay9/1 -> 1-D Lookup Table/1
  Delay8/1 -> Delay11/1
  Delay7/1 -> Delay9/1
  Delay6/1 -> Delay12/1
  Delay5/1 -> Delay13/1
  Delay4/1 -> Delay14/1
  Delay2/1 -> Delay5/1, PLSC Valid Counter/2
  Delay1/1 -> Delay4/1, PLSC Valid Counter/1
  dataIn/1 -> Delay3/1
  Product/1 -> Delay21/1
  Delay3/1 -> Delay8/1
  resetIn/1 -> Delay1/1
  Extract Bits/1 -> Delay16/1
  PLSC Valid Counter/1 -> Delay6/1, Delay7/1
  validIn/1 -> Delay2/1
  Data Type Conversion/1 -> Delay25/1
  Math Function/1 -> Delay19/1
  1-D Lookup Table/1 -> Delay10/1

== system soc_dvbs2_fpga/DVBS2/DVBS2 TxRx/DVB-S2 HDL Receiver/Synchronizer and PL Header Decoder/PL Header Recovery/PL Header Decoder/pi//2 BPSK Soft Bit Generator ==
  dataIn : Inport
  indexIndicatorIn : Inport  Port=2
  validIn : Inport  Port=3
  resetIn : Inport  Port=4
  Complex to Real-Imag : ComplexToRealImag  Output=Real
  Delay{1..12} (12 alike) : Delay
  Gain : Gain  Gain=fi(exp(1i*(3*pi/4)),1,16)  ParamDataTypeStr=Inherit: Inherit from 'Gain'  OutDataTypeStr=Inherit: Same as input
  Gain1 : Gain  Gain=fi(exp(1i*(pi/4)),1,16)  ParamDataTypeStr=Inherit: Inherit from 'Gain'  OutDataTypeStr=Inherit: Same as input
  Switch : Switch  Criteria=u2 ~= 0  SaturateOnIntegerOverflow=off  InputSameDT=off
  dataOut : Outport
  indexIndicatorOut : Outport  Port=2
  validOut : Outport  Port=3
  resetOut : Outport  Port=4
  wires:
  Delay12/1 -> resetOut/1
  Delay11/1 -> validOut/1
  Delay10/1 -> Delay12/1
  Delay9/1 -> Delay11/1
  Delay8/1 -> indexIndicatorOut/1
  Delay7/1 -> Delay8/1
  Delay6/1 -> Switch/2
  Delay5/1 -> Delay6/1
  Delay4/1 -> Switch/3
  Delay2/1 -> Switch/1
  Delay1/1 -> Gain/1
  Delay3/1 -> Gain1/1
  resetIn/1 -> Delay10/1
  Switch/1 -> Complex to Real-Imag/1
  Complex to Real-Imag/1 -> dataOut/1
  validIn/1 -> Delay9/1
  indexIndicatorIn/1 -> Delay5/1, Delay7/1
  Gain/1 -> Delay4/1
  Gain1/1 -> Delay2/1
  dataIn/1 -> Delay3/1, Delay1/1

== system soc_dvbs2_fpga/DVBS2/DVBS2 TxRx/DVB-S2 HDL Receiver/Synchronizer and PL Header Decoder/Time Frequency and Coarse Phase Synchronizer/Coarse Phase Synchronizer/Coarse Phase Corrector ==
  note: Set this value to zero to disable correction
  note: Let Z be the complex phase estimate and Xbar be the data and X be the corrected data.
      | X = Xbar * conj(Z) * (1/abs(Z))
  validIn : Inport
  dataIn : Inport  Port=2
  estimate : Inport  Port=3
  Complex to Magnitude-Angle HDL Optimized : dsphdlmathfun2/Complex to Magnitude-Angle  NumIterationsSource=Auto  NumIterations=10  OutputFormat=Magnitude  AngleFormat=Normalized  ScaleOutput=on  ScalingMethod=Shift-Add  SimulateUsing=Code generation
  Constant : Constant  Value=CPCV  OutDataTypeStr=boolean  SampleTime=-1
  Constant1 : Constant  OutMin=1  OutMax=1  OutDataTypeStr=boolean  SampleTime=-1
  Data Type Conversion : DataTypeConversion  OutDataTypeStr=fixdt(1,12,10)  SaturateOnIntegerOverflow=off  RndMeth=Floor
  Data Type Conversion2 : DataTypeConversion  OutDataTypeStr=fixdt(1,13,10)  SaturateOnIntegerOverflow=off  RndMeth=Floor
  Delay : Delay  DelayLength=15
  Delay1 : Delay  DelayLength=15
  Delay{2..4,7..8,10,13..18,22,25,28,36,38..39,41} (19 alike) : Delay  InitialCondition=0
  Delay11 : Delay  DelayLength=7  InitialCondition=0
  Delay12 : Delay  DelayLength=7  InitialCondition=0
  Delay5 : Delay  DelayLength=15
  Delay9 : Delay  DelayLength=7  InitialCondition=0
  Math Function : Math  Operator=conj  SignedPower=on  RndMeth=Zero
  Multiport Switch1 : MultiPortSwitch  DataPortOrder=Zero-based contiguous  Inputs=2  zeroidx=on  SaturateOnIntegerOverflow=off  InputSameDT=off
  Product1 : Product  OutDataTypeStr=Inherit: Same as first input
  Product2 : Product  OutDataTypeStr=Inherit: Same as first input
  Reciprocal : Subsystem  mask{WL=13, FL=10, outWL=26, Mapp=RAM - Based}
      mask prompts: WL "Input Word Length :"; FL "Input Fractional Length :"; outWL "Output Word Length :"; Mapp "Mapping Type:"
      mask init:
      | % Inverse for 18 bit numbers: partitioned into 3+15 bits. 2^3 LUTs with 2^15
      | % combinations will store a total of 2^18 combinations.
      | % As each LUT has 2^15 combinations the data type of output has a maximum
      | % limit of 32 bits (2^20 is a maximum number of bits an LUT can store)
      | 
      | % Non tunable Parameters
      | % FL = 16;
      | % outWL = 31;
      | % WL = 18;
      | % This Parameter is not given for mask
      | LUTAddrWL = WL - 1; % this will implement 2 LUTs
      | 
      | % validate Non tunable parameters
      | % condition for validation: 2^20 bits is the maximum number of bits an LUT can store
      | if LUTAddrWL >= 20   % As 2^20 is the limit
      |     error('invalid LUTAddrWL');
      | end
      | if outWL >= 2^(20-LUTAddrWL)  % 2^(20-LUTAddrWL) is the maximum outWL based on condition for validation
      |     error('invalid outWL')
      | end
      | 
      | % calculate number of LUTs required
      | muxSelectorWL = WL - LUTAddrWL;
      | nLUT = 2^muxSelectorWL;
      | 
      | % Generate all possible RWV inputs using WL and FL
      | allInputRangeSI = -2^(WL-1):2^(WL-1)-1;  % as a stored integer
      | allInputRWV = allInputRangeSI * 2^(-FL);
      | 
      | % define the function for all the RWV input
      | reciprocal = 1./allInputRWV;
      | 
      | % store the function output in LUT
      | allLUTAddr = (0:2^LUTAddrWL-1);
      | LUT = zeros(length(allLUTAddr),nLUT);
      | for i = 0:nLUT-1
      |     LUT(:,i+1) = reciprocal(i*2^LUTAddrWL+1:(i+1)*2^LUTAddrWL);
      | end
      | 
      | % quantize the function with outWL
      | NT = numerictype(fi(LUT(abs(LUT) ~= inf),1,outWL)); % inf and -inf will be quantized with max and min values with NT data type
      | if NT.WordLength < NT. FractionLength
      |     NT.FractionLength = NT.WordLength
      | end
      | LUT = fi(LUT,NT);
      | 
      | paths = find_system([gcb '/Function Impl'],'BlockType','Delay');
      | 
      | for i = 1:length(paths)
      |     if Mapp == 1
      |         hdlset_param(paths{i},'ResetType','default');
      |     else
      |         hdlset_param(paths{i},'ResetType','none');
      |     end
      | end
      mask TypeOptions Mapp: LUT - Based | RAM - Based
      mask DialogControl DescGroupVar Prompt: LUT - Based function
      mask DialogControl DescTextVar Prompt: This block is implemented for real reciprocal
      mask Display: disp(['Reciprocal\n' get_param(gcb,'Mapp') '\nLatency = 7'])
  Terminator : Terminator
  dataOut : Outport
  validOut : Outport  Port=2
  wires:
  Data Type Conversion/1 -> Complex to Magnitude-Angle HDL Optimized/1, Delay1/1
  estimate/1 -> Data Type Conversion/1
  Delay7/1 -> Delay17/1
  Delay39/1 -> Multiport Switch1/3
  Complex to Magnitude-Angle HDL Optimized/1 -> Delay10/1
  Constant1/1 -> Complex to Magnitude-Angle HDL Optimized/2
  Product1/1 -> Delay39/1
  Reciprocal/1(dataOut) -> Delay3/1
  Delay38/1 -> Delay13/1
  Delay36/1 -> Delay38/1, Product2/1
  Delay1/1 -> Delay25/1
  Delay25/1 -> Delay9/1
  Math Function/1 -> Delay28/1
  Delay28/1 -> Product2/2
  Delay16/1 -> Delay18/1
  Constant/1 -> Multiport Switch1/1
  Delay22/1 -> validOut/1
  Multiport Switch1/1 -> dataOut/1
  Product2/1 -> Delay4/1
  Delay14/1 -> Delay16/1
  Delay2/1 -> Delay12/1
  Delay5/1 -> Delay2/1
  validIn/1 -> Delay5/1
  dataIn/1 -> Delay/1
  Delay/1 -> Delay8/1
  Delay8/1 -> Delay11/1
  Delay41/1 -> Multiport Switch1/2
  Delay4/1 -> Delay15/1
  Complex to Magnitude-Angle HDL Optimized/2 -> Terminator/1
  Delay9/1 -> Math Function/1
  Delay11/1 -> Delay36/1
  Delay12/1 -> Delay14/1
  Delay10/1 -> Data Type Conversion2/1
  Delay13/1 -> Delay41/1
  Delay15/1 -> Product1/1
  Delay17/1 -> Product1/2
  Delay18/1 -> Delay22/1
  Delay3/1 -> Delay7/1
  Data Type Conversion2/1 -> Reciprocal/1(dataIn)
